simulink model "EKF"  (R2020a)
settings: Solver=VariableStepAuto  StartTime=0.0  StopTime=inf  RelTol=1e-3
libraries: robotlib x1
settings Model: Creator=johni  LastModifiedBy=johni

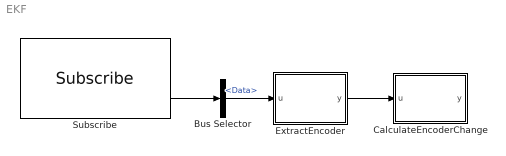
== system EKF ==
  Bus Selector : BusSelector  OutputSignals=Data
  CalculateEncoderChange : MATLAB Function  TreatAsAtomicUnit=on
  ExtractEncoder : MATLAB Function  TreatAsAtomicUnit=on
  Subscribe : robotlib/Subscribe  topicSource=Select from ROS network  topic=/zlac8015d/encoder  messageType=std_msgs/UInt32MultiArray  sampleTime=-1  messageQueueLength=1
  wires:
  Subscribe/2 -> Bus Selector/1
  Bus Selector/1 -> ExtractEncoder/1(u)  "<Data>"
  ExtractEncoder/1(y) -> CalculateEncoderChange/1(u)

== matlab function EKF/ExtractEncoder ==
  data: u input; y output
function y = fcn(u)
    
y = [u(1,:), u(2,:)];

== matlab function EKF/CalculateEncoderChange ==
  data: u input; y output
function y = fcn(u)
    
y = u;
